simulink model "PubIfDecisionTOS_MDL"  (R2020b)
settings: configuration reference "DspaceConfig" (kept outside this file)
PostLoadFcn:
  | if any(exist('dsrtsu_mdlpostloadfcn', 'file') ~= 0), dsrtsu_mdlpostloadfcn('Execute', bdroot); end
InitFcn:
  | , if any(exist('dsmpb_private', 'file') ~= 0), dsmpb_private('dsmpb_mdlclblib', 'Init', bdroot); end,
undefined symbols (not defined in the file or in its folder): C_TOS_ACCEgoRAxletoFbumplength_m, C_TOS_ACCTargetFront_Flag, C_TOS_AEBJAPedObjDxThre_Val, C_TOS_AEBJAPedObjDyThre_Val, C_TOS_AEBJATargetSize_Val, C_TOS_AEBJAVehObjDxThre_Val, C_TOS_AEBJAVehObjDyThre_Val, C_TOS_AEBJuncPedTargetSize_Val, C_TOS_AEBLatObjDxThre_Val, C_TOS_AEBLatPedDyThre_Val, C_TOS_AEBLatTargetSize_Val, C_TOS_AEBLongTargetInEgoFront_Flag, C_TOS_axAbsGround_Parameter, C_TOS_CameraConfirmedFlag, C_TOS_CNsubjWidth, C_TOS_CurrentLaneCoreMinWidth_Val, C_TOS_CutInProb_Val_Zero, C_TOS_CutOutProb_Val_Zero, C_TOS_D2R_Val, C_TOS_DefaultValueObjectToCenterLine_dy, C_TOS_EgoCarWidth_Val, C_TOS_EgoDxRefPoint_m, C_TOS_EgoRAxletoFbumplength_m, C_TOS_HalfWidthVehicle_Con, C_TOS_HWA_CurrentLaneFlag, C_TOS_HWA_LeftLaneFlag, C_TOS_HWA_MovingDir_Vaild, C_TOS_HWA_MovState_Vaild, C_TOS_HWA_RightLaneFlag, C_TOS_LaneLineCourseErrorFront, C_TOS_LaneLineCourseErrorRear, C_TOS_MotorbikeDefaultWidth_m, C_TOS_NumberOfEffectiveTargets, C_TOS_Obj_Age_Val, C_TOS_Objdx_Constraint_Val, C_TOS_ObjectDefaultWidth_m, C_TOS_ObjInCurrentLane_Val, C_TOS_ObjInCurrentLaneValid, C_TOS_ObjInLeftLaneValid, C_TOS_ObjInRightLaneValid, C_TOS_ObjNotInCurrentLane_Val, C_TOS_ObjNotREElementType, C_TOS_ObjPredictDis_dy_ConstantVal_Zeros, C_TOS_ObjToCenterLine_ConstantVal_Zeros, C_TOS_OFMObjIDInvilad_Val, C_TOS_PIL_LatDisCons_Val_zero, C_TOS_PIL_ObjectCutInFlag_b, C_TOS_PIL_ObjectCutOutFlag_b, C_TOS_PIL_ObjLaneProb_al_Val, C_TOS_PP_ObjFusType_FC_Confirm_b, C_TOS_PP_ObjFusType_FC_FR_Confirm_b, C_TOS_PP_ObjFusType_FR_Confirm_b, C_TOS_RE_80BoolDefault_Val, C_TOS_RE_80Single181Default_Val, C_TOS_RE_80Single255Default_Val, C_TOS_RE_80Uint8Default_Val, C_TOS_RE_D2R, C_TOS_RE_D_180_Val, C_TOS_RE_InvalidObjectID_Val, C_TOS_RE_InvalidTargetChainDir_Val ... (+142)
libraries: simulink x1650, TOS_LIB x361, canfdmsglib x14
(part 57 of 69)

== system PubIfDecisionTOS_MDL/TOS_20201112/TOS_2012080320/TOS/ACC/TOS_ACCLeftLane/ACC_LeftLane_Target/TOS_ACC_P4/ACC_P4_Targe/ACC_P4_Targe/TOS_ACC_ObjTypeConfirm/Subsystem1/Subsystem ==
  ObjMovState : Inport
  ACC_Target_ID_K1 : Inport  Port=2
  ACC_Target_ID_K2 : Inport  Port=3
  ACC_Target_MovState_K1 : Inport  Port=4
  ACC_Target_MovState_K2 : Inport  Port=5
  ObjectID : Inport  Port=6
  TOS_ObjMovStateCfmFlow1 : Stateflow chart  TreatAsAtomicUnit=on
  TOS_ObjMovStateCfm : Outport
  wires:
  TOS_ObjMovStateCfmFlow1/1(TOS_ObjMovStateCfm) -> TOS_ObjMovStateCfm/1
  ACC_Target_ID_K1/1 -> TOS_ObjMovStateCfmFlow1/1(ACC_TargetP0_ID_K1)
  ACC_Target_ID_K2/1 -> TOS_ObjMovStateCfmFlow1/2(ACC_TargetP0_ID_K2)
  ACC_Target_MovState_K1/1 -> TOS_ObjMovStateCfmFlow1/3(ACC_TargetP0_MovState_K1)
  ACC_Target_MovState_K2/1 -> TOS_ObjMovStateCfmFlow1/4(ACC_TargetP0_MovState_K2)
  ObjMovState/1 -> TOS_ObjMovStateCfmFlow1/5(ObjMovState)
  ObjectID/1 -> TOS_ObjMovStateCfmFlow1/6(ObjectID)

== system PubIfDecisionTOS_MDL/TOS_20201112/TOS_2012080320/TOS/ACC/TOS_ACCLeftLane/ACC_LeftLane_Target/TOS_ACC_P4/ACC_P4_Targe/ACC_P4_Targe/TOS_ACC_ObjTypeConfirm/TOS_ACCObjTypeAborDly/If Action Subsystem ==
  TOS_ACCFusionType : Inport
  Action Port : ActionPort  ActionPortLabel=else
  TOS_ACCFusionTypeFilt : Outport
  wires:
  TOS_ACCFusionType/1 -> TOS_ACCFusionTypeFilt/1

== system PubIfDecisionTOS_MDL/TOS_20201112/TOS_2012080320/TOS/ACC/TOS_ACCLeftLane/ACC_LeftLane_Target/TOS_ACC_P4/ACC_P4_Targe/ACC_P4_Targe/TOS_ACC_ObjTypeConfirm/TOS_ACCObjTypeAborDly/If Action Subsystem1 ==
  TOS_ACCFusionType : Inport
  Action Port : ActionPort  ActionPortLabel=if(u1)
  Constant : Constant  Value=0.15
  Constant4 : Constant  Value=0.05
  StateDelayAbortion : TOS_LIB/StateDelayAbortion  SystemSampleTime=-1  VariantActivationTime=update diagram  Latency=0  AutoFrameSizeCalculation=off
  TOS_ACCFusionTypeFilt : Outport
  wires:
  TOS_ACCFusionType/1 -> StateDelayAbortion/1
  Constant4/1 -> StateDelayAbortion/3
  Constant/1 -> StateDelayAbortion/2
  StateDelayAbortion/1 -> TOS_ACCFusionTypeFilt/1

== system PubIfDecisionTOS_MDL/TOS_20201112/TOS_2012080320/TOS/ACC/TOS_ACCLeftLane/ACC_LeftLane_Target/TOS_ACC_P4/ACC_P4_Targe/ACC_P4_Targe/TOS_ACC_ObstacleProbConfirm/TOS_ACCObstacleProbAborDly/If Action Subsystem ==
  TOS_ACCFusionType : Inport
  Action Port : ActionPort  ActionPortLabel=else
  TOS_ACCFusionTypeFilt : Outport
  wires:
  TOS_ACCFusionType/1 -> TOS_ACCFusionTypeFilt/1

== system PubIfDecisionTOS_MDL/TOS_20201112/TOS_2012080320/TOS/ACC/TOS_ACCLeftLane/ACC_LeftLane_Target/TOS_ACC_P4/ACC_P4_Targe/ACC_P4_Targe/TOS_ACC_ObstacleProbConfirm/TOS_ACCObstacleProbAborDly/If Action Subsystem1 ==
  TOS_ACCFusionType : Inport
  Action Port : ActionPort  ActionPortLabel=if(u1)
  Constant : Constant  Value=0.15
  Constant4 : Constant  Value=0.05
  StateDelayAbortion : TOS_LIB/StateDelayAbortion  SystemSampleTime=-1  VariantActivationTime=update diagram  Latency=0  AutoFrameSizeCalculation=off
  TOS_ACCFusionTypeFilt : Outport
  wires:
  TOS_ACCFusionType/1 -> StateDelayAbortion/1
  Constant4/1 -> StateDelayAbortion/3
  Constant/1 -> StateDelayAbortion/2
  StateDelayAbortion/1 -> TOS_ACCFusionTypeFilt/1

== system PubIfDecisionTOS_MDL/TOS_20201112/TOS_2012080320/TOS/ACC/TOS_ACCLeftLane/ACC_LeftLane_Target/TOS_ACC_P4/ACC_P4_Targe/ACC_P4_Targe/TOS_ACC_ObstacleProbConfirm/TOS_ACCObstacleProbAborDly/Subsystem ==
  ACC_TargetP0_ID_K1 : Inport
  ObjectID : Inport  Port=2
  Relational Operator : RelationalOperator  Operator===  OutDataTypeStr=boolean  RndMeth=Simplest
  ACC_SameTargetP0 : Outport
  wires:
  ACC_TargetP0_ID_K1/1 -> Relational Operator/1
  Relational Operator/1 -> ACC_SameTargetP0/1
  ObjectID/1 -> Relational Operator/2

== system PubIfDecisionTOS_MDL/TOS_20201112/TOS_2012080320/TOS/ACC/TOS_ACCLeftLane/ACC_LeftLane_Target/TOS_ACC_P4/ACC_P4_Targe/ACC_P4_Targe/TOS_ACC_TargetMovingDirConfirm/TOS_ACCMovingDirAborDly/If Action Subsystem ==
  TOS_ACCMovingDir : Inport
  Action Port : ActionPort  ActionPortLabel=else
  TOS_ACCMovingDirFilt : Outport
  wires:
  TOS_ACCMovingDir/1 -> TOS_ACCMovingDirFilt/1

== system PubIfDecisionTOS_MDL/TOS_20201112/TOS_2012080320/TOS/ACC/TOS_ACCLeftLane/ACC_LeftLane_Target/TOS_ACC_P4/ACC_P4_Targe/ACC_P4_Targe/TOS_ACC_TargetMovingDirConfirm/TOS_ACCMovingDirAborDly/If Action Subsystem1 ==
  TOS_ACCMovingDir : Inport
  Action Port : ActionPort  ActionPortLabel=if(u1)
  Constant : Constant  Value=0.15
  Constant4 : Constant  Value=0.05
  StateDelayAbortion : TOS_LIB/StateDelayAbortion  SystemSampleTime=-1  VariantActivationTime=update diagram  Latency=0  AutoFrameSizeCalculation=off
  TOS_ACCMovingDirFilt : Outport
  wires:
  TOS_ACCMovingDir/1 -> StateDelayAbortion/1
  Constant4/1 -> StateDelayAbortion/3
  Constant/1 -> StateDelayAbortion/2
  StateDelayAbortion/1 -> TOS_ACCMovingDirFilt/1

== system PubIfDecisionTOS_MDL/TOS_20201112/TOS_2012080320/TOS/ACC/TOS_ACCLeftLane/ACC_LeftLane_Target/TOS_ACC_P4/ACC_P4_Targe/ACC_P4_Targe/TOS_ACC_TargetMovingDirConfirm/TOS_ACCMovingDirAborDly/Subsystem ==
  ACC_TargetP0_ID_K1 : Inport
  ObjectID : Inport  Port=2
  Relational Operator : RelationalOperator  Operator===  OutDataTypeStr=boolean  RndMeth=Simplest
  ACC_SameTargetP0 : Outport
  wires:
  ACC_TargetP0_ID_K1/1 -> Relational Operator/1
  Relational Operator/1 -> ACC_SameTargetP0/1
  ObjectID/1 -> Relational Operator/2

== system PubIfDecisionTOS_MDL/TOS_20201112/TOS_2012080320/TOS/ACC/TOS_ACCRightLane/ACC_LeftLane_Target/TOS_ACC_P3/ACC_P3_Targe/ACC_P3_Targe/TOS_ACC_FusionTypeConfirm/TOS_ACCFusionTypeAborDly/If Action Subsystem ==
  TOS_ACCFusionType : Inport
  Action Port : ActionPort  ActionPortLabel=else
  TOS_ACCFusionTypeFilt : Outport
  wires:
  TOS_ACCFusionType/1 -> TOS_ACCFusionTypeFilt/1

== system PubIfDecisionTOS_MDL/TOS_20201112/TOS_2012080320/TOS/ACC/TOS_ACCRightLane/ACC_LeftLane_Target/TOS_ACC_P3/ACC_P3_Targe/ACC_P3_Targe/TOS_ACC_FusionTypeConfirm/TOS_ACCFusionTypeAborDly/If Action Subsystem1 ==
  TOS_ACCFusionType : Inport
  Action Port : ActionPort  ActionPortLabel=if(u1)
  Constant : Constant  Value=0.15
  Constant4 : Constant  Value=0.05
  StateDelayAbortion : TOS_LIB/StateDelayAbortion  SystemSampleTime=-1  VariantActivationTime=update diagram  Latency=0  AutoFrameSizeCalculation=off
  TOS_ACCFusionTypeFilt : Outport
  wires:
  StateDelayAbortion/1 -> TOS_ACCFusionTypeFilt/1
  Constant/1 -> StateDelayAbortion/2
  Constant4/1 -> StateDelayAbortion/3
  TOS_ACCFusionType/1 -> StateDelayAbortion/1

== system PubIfDecisionTOS_MDL/TOS_20201112/TOS_2012080320/TOS/ACC/TOS_ACCRightLane/ACC_LeftLane_Target/TOS_ACC_P3/ACC_P3_Targe/ACC_P3_Targe/TOS_ACC_ObjTypeConfirm/Subsystem1/Subsystem ==
  ObjMovState : Inport
  ACC_Target_ID_K1 : Inport  Port=2
  ACC_Target_ID_K2 : Inport  Port=3
  ACC_Target_MovState_K1 : Inport  Port=4
  ACC_Target_MovState_K2 : Inport  Port=5
  ObjectID : Inport  Port=6
  TOS_ObjMovStateCfmFlow1 : Stateflow chart  TreatAsAtomicUnit=on
  TOS_ObjMovStateCfm : Outport
  wires:
  ObjectID/1 -> TOS_ObjMovStateCfmFlow1/6(ObjectID)
  ObjMovState/1 -> TOS_ObjMovStateCfmFlow1/5(ObjMovState)
  ACC_Target_MovState_K2/1 -> TOS_ObjMovStateCfmFlow1/4(ACC_TargetP0_MovState_K2)
  ACC_Target_MovState_K1/1 -> TOS_ObjMovStateCfmFlow1/3(ACC_TargetP0_MovState_K1)
  ACC_Target_ID_K2/1 -> TOS_ObjMovStateCfmFlow1/2(ACC_TargetP0_ID_K2)
  ACC_Target_ID_K1/1 -> TOS_ObjMovStateCfmFlow1/1(ACC_TargetP0_ID_K1)
  TOS_ObjMovStateCfmFlow1/1(TOS_ObjMovStateCfm) -> TOS_ObjMovStateCfm/1

== system PubIfDecisionTOS_MDL/TOS_20201112/TOS_2012080320/TOS/ACC/TOS_ACCRightLane/ACC_LeftLane_Target/TOS_ACC_P3/ACC_P3_Targe/ACC_P3_Targe/TOS_ACC_ObjTypeConfirm/TOS_ACCObjTypeAborDly/If Action Subsystem ==
  TOS_ACCFusionType : Inport
  Action Port : ActionPort  ActionPortLabel=else
  TOS_ACCFusionTypeFilt : Outport
  wires:
  TOS_ACCFusionType/1 -> TOS_ACCFusionTypeFilt/1

== system PubIfDecisionTOS_MDL/TOS_20201112/TOS_2012080320/TOS/ACC/TOS_ACCRightLane/ACC_LeftLane_Target/TOS_ACC_P3/ACC_P3_Targe/ACC_P3_Targe/TOS_ACC_ObjTypeConfirm/TOS_ACCObjTypeAborDly/If Action Subsystem1 ==
  TOS_ACCFusionType : Inport
  Action Port : ActionPort  ActionPortLabel=if(u1)
  Constant : Constant  Value=0.15
  Constant4 : Constant  Value=0.05
  StateDelayAbortion : TOS_LIB/StateDelayAbortion  SystemSampleTime=-1  VariantActivationTime=update diagram  Latency=0  AutoFrameSizeCalculation=off
  TOS_ACCFusionTypeFilt : Outport
  wires:
  StateDelayAbortion/1 -> TOS_ACCFusionTypeFilt/1
  Constant/1 -> StateDelayAbortion/2
  Constant4/1 -> StateDelayAbortion/3
  TOS_ACCFusionType/1 -> StateDelayAbortion/1

== system PubIfDecisionTOS_MDL/TOS_20201112/TOS_2012080320/TOS/ACC/TOS_ACCRightLane/ACC_LeftLane_Target/TOS_ACC_P3/ACC_P3_Targe/ACC_P3_Targe/TOS_ACC_ObstacleProbConfirm/TOS_ACCObstacleProbAborDly/If Action Subsystem ==
  TOS_ACCFusionType : Inport
  Action Port : ActionPort  ActionPortLabel=else
  TOS_ACCFusionTypeFilt : Outport
  wires:
  TOS_ACCFusionType/1 -> TOS_ACCFusionTypeFilt/1

== system PubIfDecisionTOS_MDL/TOS_20201112/TOS_2012080320/TOS/ACC/TOS_ACCRightLane/ACC_LeftLane_Target/TOS_ACC_P3/ACC_P3_Targe/ACC_P3_Targe/TOS_ACC_ObstacleProbConfirm/TOS_ACCObstacleProbAborDly/If Action Subsystem1 ==
  TOS_ACCFusionType : Inport
  Action Port : ActionPort  ActionPortLabel=if(u1)
  Constant : Constant  Value=0.15
  Constant4 : Constant  Value=0.05
  StateDelayAbortion : TOS_LIB/StateDelayAbortion  SystemSampleTime=-1  VariantActivationTime=update diagram  Latency=0  AutoFrameSizeCalculation=off
  TOS_ACCFusionTypeFilt : Outport
  wires:
  StateDelayAbortion/1 -> TOS_ACCFusionTypeFilt/1
  Constant/1 -> StateDelayAbortion/2
  Constant4/1 -> StateDelayAbortion/3
  TOS_ACCFusionType/1 -> StateDelayAbortion/1

== system PubIfDecisionTOS_MDL/TOS_20201112/TOS_2012080320/TOS/ACC/TOS_ACCRightLane/ACC_LeftLane_Target/TOS_ACC_P3/ACC_P3_Targe/ACC_P3_Targe/TOS_ACC_ObstacleProbConfirm/TOS_ACCObstacleProbAborDly/Subsystem ==
  ACC_TargetP0_ID_K1 : Inport
  ObjectID : Inport  Port=2
  Relational Operator : RelationalOperator  Operator===  OutDataTypeStr=boolean  RndMeth=Simplest
  ACC_SameTargetP0 : Outport
  wires:
  ObjectID/1 -> Relational Operator/2
  Relational Operator/1 -> ACC_SameTargetP0/1
  ACC_TargetP0_ID_K1/1 -> Relational Operator/1

== system PubIfDecisionTOS_MDL/TOS_20201112/TOS_2012080320/TOS/ACC/TOS_ACCRightLane/ACC_LeftLane_Target/TOS_ACC_P3/ACC_P3_Targe/ACC_P3_Targe/TOS_ACC_TargetMovingDirConfirm/TOS_ACCMovingDirAborDly/If Action Subsystem ==
  TOS_ACCMovingDir : Inport
  Action Port : ActionPort  ActionPortLabel=else
  TOS_ACCMovingDirFilt : Outport
  wires:
  TOS_ACCMovingDir/1 -> TOS_ACCMovingDirFilt/1

== system PubIfDecisionTOS_MDL/TOS_20201112/TOS_2012080320/TOS/ACC/TOS_ACCRightLane/ACC_LeftLane_Target/TOS_ACC_P3/ACC_P3_Targe/ACC_P3_Targe/TOS_ACC_TargetMovingDirConfirm/TOS_ACCMovingDirAborDly/If Action Subsystem1 ==
  TOS_ACCMovingDir : Inport
  Action Port : ActionPort  ActionPortLabel=if(u1)
  Constant : Constant  Value=0.15
  Constant4 : Constant  Value=0.05
  StateDelayAbortion : TOS_LIB/StateDelayAbortion  SystemSampleTime=-1  VariantActivationTime=update diagram  Latency=0  AutoFrameSizeCalculation=off
  TOS_ACCMovingDirFilt : Outport
  wires:
  StateDelayAbortion/1 -> TOS_ACCMovingDirFilt/1
  Constant/1 -> StateDelayAbortion/2
  Constant4/1 -> StateDelayAbortion/3
  TOS_ACCMovingDir/1 -> StateDelayAbortion/1

== system PubIfDecisionTOS_MDL/TOS_20201112/TOS_2012080320/TOS/ACC/TOS_ACCRightLane/ACC_LeftLane_Target/TOS_ACC_P3/ACC_P3_Targe/ACC_P3_Targe/TOS_ACC_TargetMovingDirConfirm/TOS_ACCMovingDirAborDly/Subsystem ==
  ACC_TargetP0_ID_K1 : Inport
  ObjectID : Inport  Port=2
  Relational Operator : RelationalOperator  Operator===  OutDataTypeStr=boolean  RndMeth=Simplest
  ACC_SameTargetP0 : Outport
  wires:
  ObjectID/1 -> Relational Operator/2
  Relational Operator/1 -> ACC_SameTargetP0/1
  ACC_TargetP0_ID_K1/1 -> Relational Operator/1

== system PubIfDecisionTOS_MDL/TOS_20201112/TOS_2012080320/TOS/ACC/TOS_ACCRightLane/ACC_LeftLane_Target/TOS_ACC_P5/ACC_P5_Targe/ACC_P5_Targe/TOS_ACC_FusionTypeConfirm/TOS_ACCFusionTypeAborDly/If Action Subsystem ==
  TOS_ACCFusionType : Inport
  Action Port : ActionPort  ActionPortLabel=else
  TOS_ACCFusionTypeFilt : Outport
  wires:
  TOS_ACCFusionType/1 -> TOS_ACCFusionTypeFilt/1

== system PubIfDecisionTOS_MDL/TOS_20201112/TOS_2012080320/TOS/ACC/TOS_ACCRightLane/ACC_LeftLane_Target/TOS_ACC_P5/ACC_P5_Targe/ACC_P5_Targe/TOS_ACC_FusionTypeConfirm/TOS_ACCFusionTypeAborDly/If Action Subsystem1 ==
  TOS_ACCFusionType : Inport
  Action Port : ActionPort  ActionPortLabel=if(u1)
  Constant : Constant  Value=0.15
  Constant4 : Constant  Value=0.05
  StateDelayAbortion : TOS_LIB/StateDelayAbortion  SystemSampleTime=-1  VariantActivationTime=update diagram  Latency=0  AutoFrameSizeCalculation=off
  TOS_ACCFusionTypeFilt : Outport
  wires:
  TOS_ACCFusionType/1 -> StateDelayAbortion/1
  Constant4/1 -> StateDelayAbortion/3
  Constant/1 -> StateDelayAbortion/2
  StateDelayAbortion/1 -> TOS_ACCFusionTypeFilt/1

== system PubIfDecisionTOS_MDL/TOS_20201112/TOS_2012080320/TOS/ACC/TOS_ACCRightLane/ACC_LeftLane_Target/TOS_ACC_P5/ACC_P5_Targe/ACC_P5_Targe/TOS_ACC_ObjTypeConfirm/Subsystem1/Subsystem ==
  ObjMovState : Inport
  ACC_Target_ID_K1 : Inport  Port=2
  ACC_Target_ID_K2 : Inport  Port=3
  ACC_Target_MovState_K1 : Inport  Port=4
  ACC_Target_MovState_K2 : Inport  Port=5
  ObjectID : Inport  Port=6
  TOS_ObjMovStateCfmFlow1 : Stateflow chart  TreatAsAtomicUnit=on
  TOS_ObjMovStateCfm : Outport
  wires:
  TOS_ObjMovStateCfmFlow1/1(TOS_ObjMovStateCfm) -> TOS_ObjMovStateCfm/1
  ACC_Target_ID_K1/1 -> TOS_ObjMovStateCfmFlow1/1(ACC_TargetP0_ID_K1)
  ACC_Target_ID_K2/1 -> TOS_ObjMovStateCfmFlow1/2(ACC_TargetP0_ID_K2)
  ACC_Target_MovState_K1/1 -> TOS_ObjMovStateCfmFlow1/3(ACC_TargetP0_MovState_K1)
  ACC_Target_MovState_K2/1 -> TOS_ObjMovStateCfmFlow1/4(ACC_TargetP0_MovState_K2)
  ObjMovState/1 -> TOS_ObjMovStateCfmFlow1/5(ObjMovState)
  ObjectID/1 -> TOS_ObjMovStateCfmFlow1/6(ObjectID)

== system PubIfDecisionTOS_MDL/TOS_20201112/TOS_2012080320/TOS/ACC/TOS_ACCRightLane/ACC_LeftLane_Target/TOS_ACC_P5/ACC_P5_Targe/ACC_P5_Targe/TOS_ACC_ObjTypeConfirm/TOS_ACCObjTypeAborDly/If Action Subsystem ==
  TOS_ACCFusionType : Inport
  Action Port : ActionPort  ActionPortLabel=else
  TOS_ACCFusionTypeFilt : Outport
  wires:
  TOS_ACCFusionType/1 -> TOS_ACCFusionTypeFilt/1

== system PubIfDecisionTOS_MDL/TOS_20201112/TOS_2012080320/TOS/ACC/TOS_ACCRightLane/ACC_LeftLane_Target/TOS_ACC_P5/ACC_P5_Targe/ACC_P5_Targe/TOS_ACC_ObjTypeConfirm/TOS_ACCObjTypeAborDly/If Action Subsystem1 ==
  TOS_ACCFusionType : Inport
  Action Port : ActionPort  ActionPortLabel=if(u1)
  Constant : Constant  Value=0.15
  Constant4 : Constant  Value=0.05
  StateDelayAbortion : TOS_LIB/StateDelayAbortion  SystemSampleTime=-1  VariantActivationTime=update diagram  Latency=0  AutoFrameSizeCalculation=off
  TOS_ACCFusionTypeFilt : Outport
  wires:
  TOS_ACCFusionType/1 -> StateDelayAbortion/1
  Constant4/1 -> StateDelayAbortion/3
  Constant/1 -> StateDelayAbortion/2
  StateDelayAbortion/1 -> TOS_ACCFusionTypeFilt/1

== system PubIfDecisionTOS_MDL/TOS_20201112/TOS_2012080320/TOS/ACC/TOS_ACCRightLane/ACC_LeftLane_Target/TOS_ACC_P5/ACC_P5_Targe/ACC_P5_Targe/TOS_ACC_ObstacleProbConfirm/TOS_ACCObstacleProbAborDly/If Action Subsystem ==
  TOS_ACCFusionType : Inport
  Action Port : ActionPort  ActionPortLabel=else
  TOS_ACCFusionTypeFilt : Outport
  wires:
  TOS_ACCFusionType/1 -> TOS_ACCFusionTypeFilt/1

== system PubIfDecisionTOS_MDL/TOS_20201112/TOS_2012080320/TOS/ACC/TOS_ACCRightLane/ACC_LeftLane_Target/TOS_ACC_P5/ACC_P5_Targe/ACC_P5_Targe/TOS_ACC_ObstacleProbConfirm/TOS_ACCObstacleProbAborDly/If Action Subsystem1 ==
  TOS_ACCFusionType : Inport
  Action Port : ActionPort  ActionPortLabel=if(u1)
  Constant : Constant  Value=0.15
  Constant4 : Constant  Value=0.05
  StateDelayAbortion : TOS_LIB/StateDelayAbortion  SystemSampleTime=-1  VariantActivationTime=update diagram  Latency=0  AutoFrameSizeCalculation=off
  TOS_ACCFusionTypeFilt : Outport
  wires:
  TOS_ACCFusionType/1 -> StateDelayAbortion/1
  Constant4/1 -> StateDelayAbortion/3
  Constant/1 -> StateDelayAbortion/2
  StateDelayAbortion/1 -> TOS_ACCFusionTypeFilt/1

== system PubIfDecisionTOS_MDL/TOS_20201112/TOS_2012080320/TOS/ACC/TOS_ACCRightLane/ACC_LeftLane_Target/TOS_ACC_P5/ACC_P5_Targe/ACC_P5_Targe/TOS_ACC_ObstacleProbConfirm/TOS_ACCObstacleProbAborDly/Subsystem ==
  ACC_TargetP0_ID_K1 : Inport
  ObjectID : Inport  Port=2
  Relational Operator : RelationalOperator  Operator===  OutDataTypeStr=boolean  RndMeth=Simplest
  ACC_SameTargetP0 : Outport
  wires:
  ACC_TargetP0_ID_K1/1 -> Relational Operator/1
  Relational Operator/1 -> ACC_SameTargetP0/1
  ObjectID/1 -> Relational Operator/2

== system PubIfDecisionTOS_MDL/TOS_20201112/TOS_2012080320/TOS/ACC/TOS_ACCRightLane/ACC_LeftLane_Target/TOS_ACC_P5/ACC_P5_Targe/ACC_P5_Targe/TOS_ACC_TargetMovingDirConfirm/TOS_ACCMovingDirAborDly/If Action Subsystem ==
  TOS_ACCMovingDir : Inport
  Action Port : ActionPort  ActionPortLabel=else
  TOS_ACCMovingDirFilt : Outport
  wires:
  TOS_ACCMovingDir/1 -> TOS_ACCMovingDirFilt/1

== system PubIfDecisionTOS_MDL/TOS_20201112/TOS_2012080320/TOS/ACC/TOS_ACCRightLane/ACC_LeftLane_Target/TOS_ACC_P5/ACC_P5_Targe/ACC_P5_Targe/TOS_ACC_TargetMovingDirConfirm/TOS_ACCMovingDirAborDly/If Action Subsystem1 ==
  TOS_ACCMovingDir : Inport
  Action Port : ActionPort  ActionPortLabel=if(u1)
  Constant : Constant  Value=0.15
  Constant4 : Constant  Value=0.05
  StateDelayAbortion : TOS_LIB/StateDelayAbortion  SystemSampleTime=-1  VariantActivationTime=update diagram  Latency=0  AutoFrameSizeCalculation=off
  TOS_ACCMovingDirFilt : Outport
  wires:
  TOS_ACCMovingDir/1 -> StateDelayAbortion/1
  Constant4/1 -> StateDelayAbortion/3
  Constant/1 -> StateDelayAbortion/2
  StateDelayAbortion/1 -> TOS_ACCMovingDirFilt/1

== system PubIfDecisionTOS_MDL/TOS_20201112/TOS_2012080320/TOS/ACC/TOS_ACCRightLane/ACC_LeftLane_Target/TOS_ACC_P5/ACC_P5_Targe/ACC_P5_Targe/TOS_ACC_TargetMovingDirConfirm/TOS_ACCMovingDirAborDly/Subsystem ==
  ACC_TargetP0_ID_K1 : Inport
  ObjectID : Inport  Port=2
  Relational Operator : RelationalOperator  Operator===  OutDataTypeStr=boolean  RndMeth=Simplest
  ACC_SameTargetP0 : Outport
  wires:
  ACC_TargetP0_ID_K1/1 -> Relational Operator/1
  Relational Operator/1 -> ACC_SameTargetP0/1
  ObjectID/1 -> Relational Operator/2

== system PubIfDecisionTOS_MDL/TOS_20201112/TOS_2012080320/TOS/AEB/TOS_AEBJunct1105/AEBJunc_Object_Condition/AEBJA_TargetCondition/TOS_AEBJunc_TargetsCondition/AEBJunc_PedTargetCondition/AEBJunc_PedTargetObjectTypeFlag/AEBJunc_PedTargetObjectTypeAborDly/If Action Subsystem ==
  TOS_AEBJunc_PedObjectType : Inport
  Action Port : ActionPort
  TOS_AEBJunc_PedObjectTypeFilt : Outport
  wires:
  TOS_AEBJunc_PedObjectType/1 -> TOS_AEBJunc_PedObjectTypeFilt/1

== system PubIfDecisionTOS_MDL/TOS_20201112/TOS_2012080320/TOS/AEB/TOS_AEBJunct1105/AEBJunc_Object_Condition/AEBJA_TargetCondition/TOS_AEBJunc_TargetsCondition/AEBJunc_PedTargetCondition/AEBJunc_PedTargetObjectTypeFlag/AEBJunc_PedTargetObjectTypeAborDly/If Action Subsystem1 ==
  TOS_AEBJunc_PedObjectType : Inport
  Action Port : ActionPort
  Constant : Constant  Value=0.15
  Constant4 : Constant  Value=0.05
  StateDelayAbortion : TOS_LIB/StateDelayAbortion  SystemSampleTime=-1  VariantActivationTime=update diagram  Latency=0  AutoFrameSizeCalculation=off
  TOS_AEBJunc_PedObjectTypeFilt : Outport
  wires:
  TOS_AEBJunc_PedObjectType/1 -> StateDelayAbortion/1
  Constant4/1 -> StateDelayAbortion/3
  Constant/1 -> StateDelayAbortion/2
  StateDelayAbortion/1 -> TOS_AEBJunc_PedObjectTypeFilt/1

== system PubIfDecisionTOS_MDL/TOS_20201112/TOS_2012080320/TOS/AEB/TOS_AEBJunct1105/AEBJunc_Object_Condition/AEBJA_TargetCondition/TOS_AEBJunc_TargetsCondition/AEBJunc_PedTargetCondition/AEBJunc_PedTargetObjectTypeFlag/AEBJunc_PedTargetObjectTypeAborDly/Subsystem ==
  AEBJunc_PedTarget_ID_K1 : Inport  Partition=on  PartitionDimension=1  PartitionWidth=1  PartitionOffset=0
  ObjectID : Inport  Port=2
  For Each : ForEach  DisableCoverage=on
  Relational Operator : RelationalOperator  Operator===  OutDataTypeStr=boolean  RndMeth=Simplest
  AEBJunc_PedSameTarget : Outport  ConcatenationDimension=1
  wires:
  AEBJunc_PedTarget_ID_K1/1 -> Relational Operator/1
  Relational Operator/1 -> AEBJunc_PedSameTarget/1
  ObjectID/1 -> Relational Operator/2

== system PubIfDecisionTOS_MDL/TOS_20201112/TOS_2012080320/TOS/AEB/TOS_AEBJunct1105/AEBJunc_Object_Condition/AEBJA_TargetCondition/TOS_AEBJunc_TargetsCondition/AEBJunc_VehTargetCondition/AEBJunc_VehTargetObjectTypeFlag/AEBJunc_VehTargetObjectTypeAborDly/If Action Subsystem ==
  TOS_AEBJunc_VehObjectType : Inport
  Action Port : ActionPort
  TOS_AEBJJunc_VehObjectTypeFilt : Outport
  wires:
  TOS_AEBJunc_VehObjectType/1 -> TOS_AEBJJunc_VehObjectTypeFilt/1

== system PubIfDecisionTOS_MDL/TOS_20201112/TOS_2012080320/TOS/AEB/TOS_AEBJunct1105/AEBJunc_Object_Condition/AEBJA_TargetCondition/TOS_AEBJunc_TargetsCondition/AEBJunc_VehTargetCondition/AEBJunc_VehTargetObjectTypeFlag/AEBJunc_VehTargetObjectTypeAborDly/If Action Subsystem1 ==
  TOS_AEBJunc_VehObjectType : Inport
  Action Port : ActionPort
  Constant : Constant  Value=0.15
  Constant4 : Constant  Value=0.05
  StateDelayAbortion : TOS_LIB/StateDelayAbortion  SystemSampleTime=-1  VariantActivationTime=update diagram  Latency=0  AutoFrameSizeCalculation=off
  TOS_AEBJunc_VehObjectTypeFilt : Outport
  wires:
  TOS_AEBJunc_VehObjectType/1 -> StateDelayAbortion/1
  Constant4/1 -> StateDelayAbortion/3
  Constant/1 -> StateDelayAbortion/2
  StateDelayAbortion/1 -> TOS_AEBJunc_VehObjectTypeFilt/1

== system PubIfDecisionTOS_MDL/TOS_20201112/TOS_2012080320/TOS/AEB/TOS_AEBJunct1105/AEBJunc_Object_Condition/AEBJA_TargetCondition/TOS_AEBJunc_TargetsCondition/AEBJunc_VehTargetCondition/AEBJunc_VehTargetObjectTypeFlag/AEBJunc_VehTargetObjectTypeAborDly/Subsystem ==
  AEBJunc_VehTarget_ID_K1 : Inport  Partition=on  PartitionDimension=1  PartitionWidth=1  PartitionOffset=0
  ObjectID : Inport  Port=2
  For Each : ForEach  DisableCoverage=on
  Relational Operator : RelationalOperator  Operator===  OutDataTypeStr=boolean  RndMeth=Simplest
  AEBJunc_VehSameTarget : Outport  ConcatenationDimension=1
  wires:
  AEBJunc_VehTarget_ID_K1/1 -> Relational Operator/1
  Relational Operator/1 -> AEBJunc_VehSameTarget/1
  ObjectID/1 -> Relational Operator/2

== system PubIfDecisionTOS_MDL/TOS_20201112/TOS_2012080320/TOS/AEB/TOS_AEBJunct1105/AEBJunc_Object_Condition1/AEBJA_TargetCondition/TOS_AEBJunc_TargetsCondition/AEBJunc_PedTargetCondition/AEBJunc_PedTargetObjectTypeFlag/AEBJunc_PedTargetObjectTypeAborDly/If Action Subsystem ==
  TOS_AEBJunc_PedObjectType : Inport
  Action Port : ActionPort
  TOS_AEBJunc_PedObjectTypeFilt : Outport
  wires:
  TOS_AEBJunc_PedObjectType/1 -> TOS_AEBJunc_PedObjectTypeFilt/1

== system PubIfDecisionTOS_MDL/TOS_20201112/TOS_2012080320/TOS/AEB/TOS_AEBJunct1105/AEBJunc_Object_Condition1/AEBJA_TargetCondition/TOS_AEBJunc_TargetsCondition/AEBJunc_PedTargetCondition/AEBJunc_PedTargetObjectTypeFlag/AEBJunc_PedTargetObjectTypeAborDly/If Action Subsystem1 ==
  TOS_AEBJunc_PedObjectType : Inport
  Action Port : ActionPort
  Constant : Constant  Value=0.15
  Constant4 : Constant  Value=0.05
  StateDelayAbortion : TOS_LIB/StateDelayAbortion  SystemSampleTime=-1  VariantActivationTime=update diagram  Latency=0  AutoFrameSizeCalculation=off
  TOS_AEBJunc_PedObjectTypeFilt : Outport
  wires:
  StateDelayAbortion/1 -> TOS_AEBJunc_PedObjectTypeFilt/1
  Constant/1 -> StateDelayAbortion/2
  Constant4/1 -> StateDelayAbortion/3
  TOS_AEBJunc_PedObjectType/1 -> StateDelayAbortion/1

== system PubIfDecisionTOS_MDL/TOS_20201112/TOS_2012080320/TOS/AEB/TOS_AEBJunct1105/AEBJunc_Object_Condition1/AEBJA_TargetCondition/TOS_AEBJunc_TargetsCondition/AEBJunc_PedTargetCondition/AEBJunc_PedTargetObjectTypeFlag/AEBJunc_PedTargetObjectTypeAborDly/Subsystem ==
  AEBJunc_PedTarget_ID_K1 : Inport  Partition=on  PartitionDimension=1  PartitionWidth=1  PartitionOffset=0
  ObjectID : Inport  Port=2
  For Each : ForEach  DisableCoverage=on
  Relational Operator : RelationalOperator  Operator===  OutDataTypeStr=boolean  RndMeth=Simplest
  AEBJunc_PedSameTarget : Outport  ConcatenationDimension=1
  wires:
  ObjectID/1 -> Relational Operator/2
  Relational Operator/1 -> AEBJunc_PedSameTarget/1
  AEBJunc_PedTarget_ID_K1/1 -> Relational Operator/1

== system PubIfDecisionTOS_MDL/TOS_20201112/TOS_2012080320/TOS/AEB/TOS_AEBJunct1105/AEBJunc_Object_Condition1/AEBJA_TargetCondition/TOS_AEBJunc_TargetsCondition/AEBJunc_VehTargetCondition/AEBJunc_VehTargetObjectTypeFlag/AEBJunc_VehTargetObjectTypeAborDly/If Action Subsystem ==
  TOS_AEBJunc_VehObjectType : Inport
  Action Port : ActionPort
  TOS_AEBJJunc_VehObjectTypeFilt : Outport
  wires:
  TOS_AEBJunc_VehObjectType/1 -> TOS_AEBJJunc_VehObjectTypeFilt/1

== system PubIfDecisionTOS_MDL/TOS_20201112/TOS_2012080320/TOS/AEB/TOS_AEBJunct1105/AEBJunc_Object_Condition1/AEBJA_TargetCondition/TOS_AEBJunc_TargetsCondition/AEBJunc_VehTargetCondition/AEBJunc_VehTargetObjectTypeFlag/AEBJunc_VehTargetObjectTypeAborDly/If Action Subsystem1 ==
  TOS_AEBJunc_VehObjectType : Inport
  Action Port : ActionPort
  Constant : Constant  Value=0.15
  Constant4 : Constant  Value=0.05
  StateDelayAbortion : TOS_LIB/StateDelayAbortion  SystemSampleTime=-1  VariantActivationTime=update diagram  Latency=0  AutoFrameSizeCalculation=off
  TOS_AEBJunc_VehObjectTypeFilt : Outport
  wires:
  StateDelayAbortion/1 -> TOS_AEBJunc_VehObjectTypeFilt/1
  Constant/1 -> StateDelayAbortion/2
  Constant4/1 -> StateDelayAbortion/3
  TOS_AEBJunc_VehObjectType/1 -> StateDelayAbortion/1

== system PubIfDecisionTOS_MDL/TOS_20201112/TOS_2012080320/TOS/AEB/TOS_AEBJunct1105/AEBJunc_Object_Condition1/AEBJA_TargetCondition/TOS_AEBJunc_TargetsCondition/AEBJunc_VehTargetCondition/AEBJunc_VehTargetObjectTypeFlag/AEBJunc_VehTargetObjectTypeAborDly/Subsystem ==
  AEBJunc_VehTarget_ID_K1 : Inport  Partition=on  PartitionDimension=1  PartitionWidth=1  PartitionOffset=0
  ObjectID : Inport  Port=2
  For Each : ForEach  DisableCoverage=on
  Relational Operator : RelationalOperator  Operator===  OutDataTypeStr=boolean  RndMeth=Simplest
  AEBJunc_VehSameTarget : Outport  ConcatenationDimension=1
  wires:
  ObjectID/1 -> Relational Operator/2
  Relational Operator/1 -> AEBJunc_VehSameTarget/1
  AEBJunc_VehTarget_ID_K1/1 -> Relational Operator/1

== system PubIfDecisionTOS_MDL/TOS_20201112/TOS_2012080320/TOS/AEB/TOS_AEBJunct_20201208/AEBJunc_Object_Condition/AEBJA_TargetCondition/TOS_AEBJunc_TargetsCondition/AEBJunc_PedTargetCondition/AEBJunc_PedTargetMoveDir/AEBLat_TargetMovDirAborDly/If Action Subsystem ==
  TOS_AEBJunc_MovDir_Flag : Inport
  Action Port : ActionPort  ActionPortLabel=else
  TOS_AEBJunc_MovDirFlag : Outport
  wires:
  TOS_AEBJunc_MovDir_Flag/1 -> TOS_AEBJunc_MovDirFlag/1

== system PubIfDecisionTOS_MDL/TOS_20201112/TOS_2012080320/TOS/AEB/TOS_AEBJunct_20201208/AEBJunc_Object_Condition/AEBJA_TargetCondition/TOS_AEBJunc_TargetsCondition/AEBJunc_PedTargetCondition/AEBJunc_PedTargetMoveDir/AEBLat_TargetMovDirAborDly/If Action Subsystem1 ==
  TOS_AEBJunc_MovDir_Flag : Inport
  Action Port : ActionPort  ActionPortLabel=if(u1)
  Constant : Constant  Value=0.15
  Constant4 : Constant  Value=0.05
  StateDelayAbortion : TOS_LIB/StateDelayAbortion  SystemSampleTime=-1  VariantActivationTime=update diagram  Latency=0  AutoFrameSizeCalculation=off
  TOS_AEBJunc_MovDirFlag_Delay : Outport
  wires:
  TOS_AEBJunc_MovDir_Flag/1 -> StateDelayAbortion/1
  Constant4/1 -> StateDelayAbortion/3
  Constant/1 -> StateDelayAbortion/2
  StateDelayAbortion/1 -> TOS_AEBJunc_MovDirFlag_Delay/1

== system PubIfDecisionTOS_MDL/TOS_20201112/TOS_2012080320/TOS/AEB/TOS_AEBJunct_20201208/AEBJunc_Object_Condition/AEBJA_TargetCondition/TOS_AEBJunc_TargetsCondition/AEBJunc_PedTargetCondition/AEBJunc_PedTargetMoveDir/AEBLat_TargetMovDirAborDly/Subsystem ==
  AEBJunc_Target_ID_K1 : Inport  Partition=on  PartitionDimension=1  PartitionWidth=1  PartitionOffset=0
  ObjectID : Inport  Port=2
  For Each : ForEach  DisableCoverage=on
  Relational Operator : RelationalOperator  Operator===  OutDataTypeStr=boolean  RndMeth=Simplest
  AEBJunc_SameTarget : Outport  ConcatenationDimension=1
  wires:
  AEBJunc_Target_ID_K1/1 -> Relational Operator/1
  ObjectID/1 -> Relational Operator/2
  Relational Operator/1 -> AEBJunc_SameTarget/1

== system PubIfDecisionTOS_MDL/TOS_20201112/TOS_2012080320/TOS/AEB/TOS_AEBJunct_20201208/AEBJunc_Object_Condition/AEBJA_TargetCondition/TOS_AEBJunc_TargetsCondition/AEBJunc_PedTargetCondition/AEBJunc_PedTargetObjectTypeFlag/AEBJunc_PedTargetObjectTypeAborDly/If Action Subsystem ==
  TOS_AEBJunc_PedObjectType : Inport
  Action Port : ActionPort  ActionPortLabel=else
  TOS_AEBJunc_PedObjectTypeFilt : Outport
  wires:
  TOS_AEBJunc_PedObjectType/1 -> TOS_AEBJunc_PedObjectTypeFilt/1

== system PubIfDecisionTOS_MDL/TOS_20201112/TOS_2012080320/TOS/AEB/TOS_AEBJunct_20201208/AEBJunc_Object_Condition/AEBJA_TargetCondition/TOS_AEBJunc_TargetsCondition/AEBJunc_PedTargetCondition/AEBJunc_PedTargetObjectTypeFlag/AEBJunc_PedTargetObjectTypeAborDly/If Action Subsystem1 ==
  TOS_AEBJunc_PedObjectType : Inport
  Action Port : ActionPort  ActionPortLabel=if(u1)
  Constant : Constant  Value=0.15
  Constant4 : Constant  Value=0.05
  StateDelayAbortion : TOS_LIB/StateDelayAbortion  SystemSampleTime=-1  VariantActivationTime=update diagram  Latency=0  AutoFrameSizeCalculation=off
  TOS_AEBJunc_PedObjectTypeFilt : Outport
  wires:
  TOS_AEBJunc_PedObjectType/1 -> StateDelayAbortion/1
  Constant4/1 -> StateDelayAbortion/3
  Constant/1 -> StateDelayAbortion/2
  StateDelayAbortion/1 -> TOS_AEBJunc_PedObjectTypeFilt/1

== system PubIfDecisionTOS_MDL/TOS_20201112/TOS_2012080320/TOS/AEB/TOS_AEBJunct_20201208/AEBJunc_Object_Condition/AEBJA_TargetCondition/TOS_AEBJunc_TargetsCondition/AEBJunc_PedTargetCondition/AEBJunc_PedTargetObjectTypeFlag/AEBJunc_PedTargetObjectTypeAborDly/Subsystem ==
  AEBJunc_PedTarget_ID_K1 : Inport  Partition=on  PartitionDimension=1  PartitionWidth=1  PartitionOffset=0
  ObjectID : Inport  Port=2
  For Each : ForEach  DisableCoverage=on
  Relational Operator : RelationalOperator  Operator===  OutDataTypeStr=boolean  RndMeth=Simplest
  AEBJunc_PedSameTarget : Outport  ConcatenationDimension=1
  wires:
  AEBJunc_PedTarget_ID_K1/1 -> Relational Operator/1
  Relational Operator/1 -> AEBJunc_PedSameTarget/1
  ObjectID/1 -> Relational Operator/2

== system PubIfDecisionTOS_MDL/TOS_20201112/TOS_2012080320/TOS/AEB/TOS_AEBJunct_20201208/AEBJunc_Object_Condition/AEBJA_TargetCondition/TOS_AEBJunc_TargetsCondition/AEBJunc_VehTargetCondition/AEBJunc_VehTargetObjectTypeFlag/AEBJunc_VehTargetObjectTypeAborDly/If Action Subsystem ==
  TOS_AEBJunc_VehObjectType : Inport
  Action Port : ActionPort  ActionPortLabel=else
  TOS_AEBJJunc_VehObjectTypeFilt : Outport
  wires:
  TOS_AEBJunc_VehObjectType/1 -> TOS_AEBJJunc_VehObjectTypeFilt/1

== system PubIfDecisionTOS_MDL/TOS_20201112/TOS_2012080320/TOS/AEB/TOS_AEBJunct_20201208/AEBJunc_Object_Condition/AEBJA_TargetCondition/TOS_AEBJunc_TargetsCondition/AEBJunc_VehTargetCondition/AEBJunc_VehTargetObjectTypeFlag/AEBJunc_VehTargetObjectTypeAborDly/If Action Subsystem1 ==
  TOS_AEBJunc_VehObjectType : Inport
  Action Port : ActionPort  ActionPortLabel=if(u1)
  Constant : Constant  Value=0.15
  Constant4 : Constant  Value=0.05
  StateDelayAbortion : TOS_LIB/StateDelayAbortion  SystemSampleTime=-1  VariantActivationTime=update diagram  Latency=0  AutoFrameSizeCalculation=off
  TOS_AEBJunc_VehObjectTypeFilt : Outport
  wires:
  TOS_AEBJunc_VehObjectType/1 -> StateDelayAbortion/1
  Constant4/1 -> StateDelayAbortion/3
  Constant/1 -> StateDelayAbortion/2
  StateDelayAbortion/1 -> TOS_AEBJunc_VehObjectTypeFilt/1

== system PubIfDecisionTOS_MDL/TOS_20201112/TOS_2012080320/TOS/AEB/TOS_AEBJunct_20201208/AEBJunc_Object_Condition/AEBJA_TargetCondition/TOS_AEBJunc_TargetsCondition/AEBJunc_VehTargetCondition/AEBJunc_VehTargetObjectTypeFlag/AEBJunc_VehTargetObjectTypeAborDly/Subsystem ==
  AEBJunc_VehTarget_ID_K1 : Inport  Partition=on  PartitionDimension=1  PartitionWidth=1  PartitionOffset=0
  ObjectID : Inport  Port=2
  For Each : ForEach  DisableCoverage=on
  Relational Operator : RelationalOperator  Operator===  OutDataTypeStr=boolean  RndMeth=Simplest
  AEBJunc_VehSameTarget : Outport  ConcatenationDimension=1
  wires:
  AEBJunc_VehTarget_ID_K1/1 -> Relational Operator/1
  Relational Operator/1 -> AEBJunc_VehSameTarget/1
  ObjectID/1 -> Relational Operator/2

== system PubIfDecisionTOS_MDL/TOS_20201112/TOS_2012080320/TOS/AEB/TOS_AEBJunct_20201208/AEBJunc_Object_Condition/AEBJA_TargetCondition/TOS_AEBJunc_TargetsCondition/AEBJunc_VehTargetCondition/TOS_AEBJunc_VehTargetMoveDir/AEBJunc_TargetMovDirAborDly/If Action Subsystem ==
  TOS_AEBJunc_MovDir_Flag : Inport
  Action Port : ActionPort  ActionPortLabel=else
  TOS_AEBJunc_MovDirFlag : Outport
  wires:
  TOS_AEBJunc_MovDir_Flag/1 -> TOS_AEBJunc_MovDirFlag/1

== system PubIfDecisionTOS_MDL/TOS_20201112/TOS_2012080320/TOS/AEB/TOS_AEBJunct_20201208/AEBJunc_Object_Condition/AEBJA_TargetCondition/TOS_AEBJunc_TargetsCondition/AEBJunc_VehTargetCondition/TOS_AEBJunc_VehTargetMoveDir/AEBJunc_TargetMovDirAborDly/If Action Subsystem1 ==
  TOS_AEBJunc_MovDir_Flag : Inport
  Action Port : ActionPort  ActionPortLabel=if(u1)
  Constant : Constant  Value=0.15
  Constant4 : Constant  Value=0.05
  StateDelayAbortion : TOS_LIB/StateDelayAbortion  SystemSampleTime=-1  VariantActivationTime=update diagram  Latency=0  AutoFrameSizeCalculation=off
  TOS_AEBJunc_MovDirFlag_Delay : Outport
  wires:
  TOS_AEBJunc_MovDir_Flag/1 -> StateDelayAbortion/1
  Constant4/1 -> StateDelayAbortion/3
  Constant/1 -> StateDelayAbortion/2
  StateDelayAbortion/1 -> TOS_AEBJunc_MovDirFlag_Delay/1

== system PubIfDecisionTOS_MDL/TOS_20201112/TOS_2012080320/TOS/AEB/TOS_AEBJunct_20201208/AEBJunc_Object_Condition/AEBJA_TargetCondition/TOS_AEBJunc_TargetsCondition/AEBJunc_VehTargetCondition/TOS_AEBJunc_VehTargetMoveDir/AEBJunc_TargetMovDirAborDly/Subsystem ==
  AEBJunc_Target_ID_K1 : Inport  Partition=on  PartitionDimension=1  PartitionWidth=1  PartitionOffset=0
  ObjectID : Inport  Port=2
  For Each : ForEach  DisableCoverage=on
  Relational Operator : RelationalOperator  Operator===  OutDataTypeStr=boolean  RndMeth=Simplest
  AEBJunc_SameTarget : Outport  ConcatenationDimension=1
  wires:
  AEBJunc_Target_ID_K1/1 -> Relational Operator/1
  ObjectID/1 -> Relational Operator/2
  Relational Operator/1 -> AEBJunc_SameTarget/1

== system PubIfDecisionTOS_MDL/TOS_20201112/TOS_2012080320/TOS/AEB/TOS_AEBJunct_20201208/AEBJunc_Object_Condition1/AEBJA_TargetCondition/TOS_AEBJunc_TargetsCondition/AEBJunc_PedTargetCondition/AEBJunc_PedTargetObjectTypeFlag/AEBJunc_PedTargetObjectTypeAborDly/If Action Subsystem ==
  TOS_AEBJunc_PedObjectType : Inport
  Action Port : ActionPort
  TOS_AEBJunc_PedObjectTypeFilt : Outport
  wires:
  TOS_AEBJunc_PedObjectType/1 -> TOS_AEBJunc_PedObjectTypeFilt/1

== system PubIfDecisionTOS_MDL/TOS_20201112/TOS_2012080320/TOS/AEB/TOS_AEBJunct_20201208/AEBJunc_Object_Condition1/AEBJA_TargetCondition/TOS_AEBJunc_TargetsCondition/AEBJunc_PedTargetCondition/AEBJunc_PedTargetObjectTypeFlag/AEBJunc_PedTargetObjectTypeAborDly/If Action Subsystem1 ==
  TOS_AEBJunc_PedObjectType : Inport
  Action Port : ActionPort
  Constant : Constant  Value=0.15
  Constant4 : Constant  Value=0.05
  StateDelayAbortion : TOS_LIB/StateDelayAbortion  SystemSampleTime=-1  VariantActivationTime=update diagram  Latency=0  AutoFrameSizeCalculation=off
  TOS_AEBJunc_PedObjectTypeFilt : Outport
  wires:
  StateDelayAbortion/1 -> TOS_AEBJunc_PedObjectTypeFilt/1
  Constant/1 -> StateDelayAbortion/2
  Constant4/1 -> StateDelayAbortion/3
  TOS_AEBJunc_PedObjectType/1 -> StateDelayAbortion/1

== system PubIfDecisionTOS_MDL/TOS_20201112/TOS_2012080320/TOS/AEB/TOS_AEBJunct_20201208/AEBJunc_Object_Condition1/AEBJA_TargetCondition/TOS_AEBJunc_TargetsCondition/AEBJunc_PedTargetCondition/AEBJunc_PedTargetObjectTypeFlag/AEBJunc_PedTargetObjectTypeAborDly/Subsystem ==
  AEBJunc_PedTarget_ID_K1 : Inport  Partition=on  PartitionDimension=1  PartitionWidth=1  PartitionOffset=0
  ObjectID : Inport  Port=2
  For Each : ForEach  DisableCoverage=on
  Relational Operator : RelationalOperator  Operator===  OutDataTypeStr=boolean  RndMeth=Simplest
  AEBJunc_PedSameTarget : Outport  ConcatenationDimension=1
  wires:
  ObjectID/1 -> Relational Operator/2
  Relational Operator/1 -> AEBJunc_PedSameTarget/1
  AEBJunc_PedTarget_ID_K1/1 -> Relational Operator/1

== system PubIfDecisionTOS_MDL/TOS_20201112/TOS_2012080320/TOS/AEB/TOS_AEBJunct_20201208/AEBJunc_Object_Condition1/AEBJA_TargetCondition/TOS_AEBJunc_TargetsCondition/AEBJunc_VehTargetCondition/AEBJunc_VehTargetObjectTypeFlag/AEBJunc_VehTargetObjectTypeAborDly/If Action Subsystem ==
  TOS_AEBJunc_VehObjectType : Inport
  Action Port : ActionPort
  TOS_AEBJJunc_VehObjectTypeFilt : Outport
  wires:
  TOS_AEBJunc_VehObjectType/1 -> TOS_AEBJJunc_VehObjectTypeFilt/1

== system PubIfDecisionTOS_MDL/TOS_20201112/TOS_2012080320/TOS/AEB/TOS_AEBJunct_20201208/AEBJunc_Object_Condition1/AEBJA_TargetCondition/TOS_AEBJunc_TargetsCondition/AEBJunc_VehTargetCondition/AEBJunc_VehTargetObjectTypeFlag/AEBJunc_VehTargetObjectTypeAborDly/If Action Subsystem1 ==
  TOS_AEBJunc_VehObjectType : Inport
  Action Port : ActionPort
  Constant : Constant  Value=0.15
  Constant4 : Constant  Value=0.05
  StateDelayAbortion : TOS_LIB/StateDelayAbortion  SystemSampleTime=-1  VariantActivationTime=update diagram  Latency=0  AutoFrameSizeCalculation=off
  TOS_AEBJunc_VehObjectTypeFilt : Outport
  wires:
  StateDelayAbortion/1 -> TOS_AEBJunc_VehObjectTypeFilt/1
  Constant/1 -> StateDelayAbortion/2
  Constant4/1 -> StateDelayAbortion/3
  TOS_AEBJunc_VehObjectType/1 -> StateDelayAbortion/1

== system PubIfDecisionTOS_MDL/TOS_20201112/TOS_2012080320/TOS/AEB/TOS_AEBJunct_20201208/AEBJunc_Object_Condition1/AEBJA_TargetCondition/TOS_AEBJunc_TargetsCondition/AEBJunc_VehTargetCondition/AEBJunc_VehTargetObjectTypeFlag/AEBJunc_VehTargetObjectTypeAborDly/Subsystem ==
  AEBJunc_VehTarget_ID_K1 : Inport  Partition=on  PartitionDimension=1  PartitionWidth=1  PartitionOffset=0
  ObjectID : Inport  Port=2
  For Each : ForEach  DisableCoverage=on
  Relational Operator : RelationalOperator  Operator===  OutDataTypeStr=boolean  RndMeth=Simplest
  AEBJunc_VehSameTarget : Outport  ConcatenationDimension=1
  wires:
  ObjectID/1 -> Relational Operator/2
  Relational Operator/1 -> AEBJunc_VehSameTarget/1
  AEBJunc_VehTarget_ID_K1/1 -> Relational Operator/1

== system PubIfDecisionTOS_MDL/TOS_20201112/TOS_2012080320/TOS/AEB/TOS_AEBLong/AEBLong_Confirm/AEBLong/AEBLong_TrgConfirm/AEBLongTrgJudg/TOS_AEBLong_ObjFusType/TOS_ACCFusionTypeAborDly/If Action Subsystem ==
  TOS_ACCFusionType : Inport
  Action Port : ActionPort  ActionPortLabel=else
  TOS_ACCFusionTypeFilt : Outport
  wires:
  TOS_ACCFusionType/1 -> TOS_ACCFusionTypeFilt/1

== system PubIfDecisionTOS_MDL/TOS_20201112/TOS_2012080320/TOS/AEB/TOS_AEBLong/AEBLong_Confirm/AEBLong/AEBLong_TrgConfirm/AEBLongTrgJudg/TOS_AEBLong_ObjFusType/TOS_ACCFusionTypeAborDly/If Action Subsystem1 ==
  TOS_ACCFusionType : Inport
  Action Port : ActionPort  ActionPortLabel=if(u1)
  Constant : Constant  Value=0.15
  Constant4 : Constant  Value=0.05
  StateDelayAbortion : TOS_LIB/StateDelayAbortion  SystemSampleTime=-1  VariantActivationTime=update diagram  Latency=0  AutoFrameSizeCalculation=off
  TOS_ACCFusionTypeFilt : Outport
  wires:
  TOS_ACCFusionType/1 -> StateDelayAbortion/1
  Constant4/1 -> StateDelayAbortion/3
  Constant/1 -> StateDelayAbortion/2
  StateDelayAbortion/1 -> TOS_ACCFusionTypeFilt/1

== system PubIfDecisionTOS_MDL/TOS_20201112/TOS_2012080320/TOS/AEB/TOS_AEBLong/AEBLong_Confirm/AEBLong/AEBLong_TrgConfirm/AEBLongTrgJudg/TOS_AEBLong_ObstacleProb/TOS_ACCObstacleProbAborDly/If Action Subsystem ==
  TOS_AEBObstacleProb : Inport
  Action Port : ActionPort  ActionPortLabel=else
  TOS_AEBObstacleProbFilt : Outport
  wires:
  TOS_AEBObstacleProb/1 -> TOS_AEBObstacleProbFilt/1

== system PubIfDecisionTOS_MDL/TOS_20201112/TOS_2012080320/TOS/AEB/TOS_AEBLong/AEBLong_Confirm/AEBLong/AEBLong_TrgConfirm/AEBLongTrgJudg/TOS_AEBLong_ObstacleProb/TOS_ACCObstacleProbAborDly/If Action Subsystem1 ==
  TOS_AEBObstacleProb : Inport
  Action Port : ActionPort  ActionPortLabel=if(u1)
  Constant : Constant  Value=0.15
  Constant4 : Constant  Value=0.05
  StateDelayAbortion : TOS_LIB/StateDelayAbortion  SystemSampleTime=-1  VariantActivationTime=update diagram  Latency=0  AutoFrameSizeCalculation=off
  TOS_AEBObstacleProbFilt : Outport
  wires:
  TOS_AEBObstacleProb/1 -> StateDelayAbortion/1
  Constant4/1 -> StateDelayAbortion/3
  Constant/1 -> StateDelayAbortion/2
  StateDelayAbortion/1 -> TOS_AEBObstacleProbFilt/1

== system PubIfDecisionTOS_MDL/TOS_20201112/TOS_2012080320/TOS/AEB/TOS_AEBLong/AEBLong_Confirm/AEBLong/AEBLong_TrgConfirm/AEBLongTrgJudg/TOS_AEBLong_ObstacleProb/TOS_ACCObstacleProbAborDly/Subsystem ==
  AEBLong_Target_ID_K1 : Inport
  ObjectID : Inport  Port=2
  Relational Operator : RelationalOperator  Operator===  OutDataTypeStr=boolean  RndMeth=Simplest
  AEBLong_SameTargetP0 : Outport
  wires:
  AEBLong_Target_ID_K1/1 -> Relational Operator/1
  Relational Operator/1 -> AEBLong_SameTargetP0/1
  ObjectID/1 -> Relational Operator/2

== system PubIfDecisionTOS_MDL/TOS_20201112/TOS_2012080320/TOS/AEB/TOS_AEBLong/AEBLong_Confirm/AEBLong/AEBLong_TrgConfirm/AEBLongTrgJudg/TOS_AEBLong_TargetMovingDir/ObjMovingDirSignalProcessing1/MappingObjInCurveLaneVXVY ==
  LM_LR_Bus : Inport
  Bus Creator : BusCreator  Inputs=6
  Bus Selector : BusSelector  OutputSignals=Object_DX,Object_VX,Object_VY,LM_LR_Bus.LM_LR_Line01.pC1,LM_LR_Bus.LM_LR_Line01.pC2,LM_LR_Bus.LM_LR_Line01.dDisStart,LM_LR_Bus.LM_LR_Line01.dDisEnd,LM_LR_Bus.LM_LR_Line02.pC1,LM_LR_Bus.LM_LR_Line02.pC2,LM_LR_Bus.LM_LR_Line02.dDisStart,LM_LR_Bus.LM_LR_Line02.dDisEnd,LM_LR_Bus.LM_LR_Line03.pC1,LM_LR_Bus.LM_LR_Line03.pC2,LM_LR_Bus.LM_LR_Line03.dDisStart,LM_LR_Bus.LM_LR_Line03.dDisEnd,LM_LR_Bus.LM_LR_Line04.pC1,LM_LR_Bus.LM_LR_Line04.pC2,LM_LR_Bus.LM_LR_Line04.dDisStart,LM_LR_Bus.LM_LR_Line04.dDisEnd,LM_LR_Bus.LM_LR_Line05.pC1,LM_LR_Bus.LM_LR_Line05.pC2,LM_LR_Bus.LM_LR_Line05.dDisStart,LM_LR_Bus.LM_LR_Line05.dDisEnd,LM_LR_Bus.LM_LR_Line06.pC1,LM_LR_Bus.LM_LR_Line06.pC2,LM_LR_Bus.LM_LR_Line06.dDisStart,LM_LR_Bus.LM_LR_Line06.dDisEnd
  Bus Selector1 : BusSelector  OutputSignals=Object_DX,Object_DY,Object_MovingState
  ObjectInCurveLaneMappingVXVY : Subsystem
  ObjectVYVXAngle : Subsystem
  Object_LM_PartInfor : Outport
  wires:
  ObjectInCurveLaneMappingVXVY/1(Object_MappingVX) -> ObjectVYVXAngle/1(Object_MappingVX)  "Object_MappingVX"
  LM_LR_Bus/1 -> Bus Selector/1, Bus Selector1/1
  Bus Selector/3 -> ObjectInCurveLaneMappingVXVY/3(Object_VY)  "<Object_VY>"
  Bus Selector/23 -> ObjectInCurveLaneMappingVXVY/23(line05_dDisEnd)  "<dDisEnd>"
  Bus Selector/24 -> ObjectInCurveLaneMappingVXVY/24(line06_C1)  "<pC1>"
  Bus Selector/20 -> ObjectInCurveLaneMappingVXVY/20(line05_C1)  "<pC1>"
  Bus Selector/6 -> ObjectInCurveLaneMappingVXVY/6(line01_dDisStart)  "<dDisStart>"
  Bus Selector/2 -> ObjectInCurveLaneMappingVXVY/2(Object_VX)  "<Object_VX>"
  Bus Selector/11 -> ObjectInCurveLaneMappingVXVY/11(line02_dDisEnd)  "<dDisEnd>"
  Bus Selector/1 -> ObjectInCurveLaneMappingVXVY/1(Object_DX)  "<Object_DX>"
  Bus Selector/16 -> ObjectInCurveLaneMappingVXVY/16(line04_C1)  "<pC1>"
  Bus Selector/18 -> ObjectInCurveLaneMappingVXVY/18(line04_dDisStart)  "<dDisStart>"
  Bus Selector/4 -> ObjectInCurveLaneMappingVXVY/4(line01_C1)  "<pC1>"
  Bus Selector/15 -> ObjectInCurveLaneMappingVXVY/15(line03_dDisEnd)  "<dDisEnd>"
  Bus Selector/7 -> ObjectInCurveLaneMappingVXVY/7(line01_dDisEnd)  "<dDisEnd>"
  Bus Selector/10 -> ObjectInCurveLaneMappingVXVY/10(line02_dDisStart)  "<dDisStart>"
  Bus Selector/22 -> ObjectInCurveLaneMappingVXVY/22(line05_dDisStart)  "<dDisStart>"
  Bus Selector/14 -> ObjectInCurveLaneMappingVXVY/14(line03_dDisStart)  "<dDisStart>"
  Bus Selector/27 -> ObjectInCurveLaneMappingVXVY/27(line06_dDisEnd)  "<dDisEnd>"
  Bus Selector/26 -> ObjectInCurveLaneMappingVXVY/26(line06_dDisStart)  "<dDisStart>"
  Bus Selector/12 -> ObjectInCurveLaneMappingVXVY/12(line03_C1)  "<pC1>"
  Bus Selector/8 -> ObjectInCurveLaneMappingVXVY/8(line02_C1)  "<pC1>"
  Bus Selector/19 -> ObjectInCurveLaneMappingVXVY/19(line04_dDisEnd)  "<dDisEnd>"
  Bus Selector/5 -> ObjectInCurveLaneMappingVXVY/5(line01_C2)  "<pC2>"
  Bus Selector/25 -> ObjectInCurveLaneMappingVXVY/25(line06_C2)  "<pC2>"
  Bus Selector/9 -> ObjectInCurveLaneMappingVXVY/9(line02_C2)  "<pC2>"
  Bus Selector/13 -> ObjectInCurveLaneMappingVXVY/13(line03_C2)  "<pC2>"
  Bus Selector/17 -> ObjectInCurveLaneMappingVXVY/17(line04_C2)  "<pC2>"
  Bus Selector/21 -> ObjectInCurveLaneMappingVXVY/21(line05_C2)  "<pC2>"
  ObjectInCurveLaneMappingVXVY/2(Object_MappingVY) -> ObjectVYVXAngle/2(Object_MappingVY)  "Object_MappingVY"
  Bus Selector1/1 -> Bus Creator/1  "<Object_DX>"
  Bus Selector1/2 -> Bus Creator/2  "<Object_DY>"
  Bus Creator/1 -> Object_LM_PartInfor/1
  ObjectVYVXAngle/1(ObjectVYVXAngle) -> Bus Creator/4  "ObjectVYVXAngle"
  ObjectVYVXAngle/2(ObjectMappingVY) -> Bus Creator/5  "ObjectMappingVY"
  ObjectVYVXAngle/3(ObjectMappingVX) -> Bus Creator/6  "ObjectMappingVX"
  Bus Selector1/3 -> Bus Creator/3  "<Object_MovingState>"
